simulink model "linear"  (R2016b)
settings: Solver=VariableStepAuto  StartTime=0.0  StopTime=100.0  RelTol=1e-3
undefined symbols (not defined in the file or in its folder): magnitude
libraries: simulink x1
settings Model: Creator=tangxiaoli  LastModifiedBy=tangxiaoli

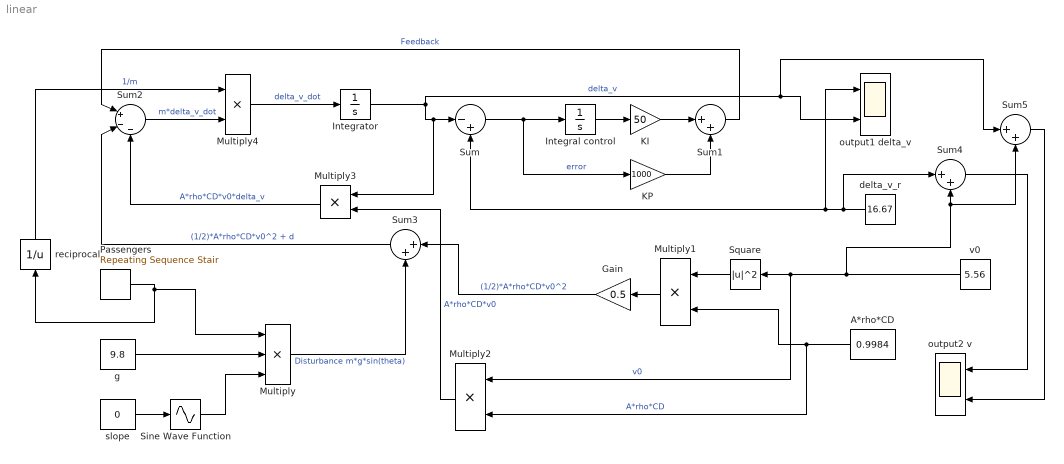
== system linear ==
  " Square" : Math  Operator=magnitude^2  SaturateOnIntegerOverflow=on
  A*rho*CD : Constant  Value=0.9984
  Gain : Gain  Gain=0.5
  Integral control : Integrator
  Integrator : Integrator
  KI : Gain  Gain=50
  KP : Gain  Gain=1000
  Multiply : Product  Inputs=***
  Multiply{1..4} (4 alike) : Product  Inputs=**
  Passengers : simulink/Sources/Repeating Sequence Stair  OutValues=[1600 1662 1724 1786 1848 1910].'  tsamp=20  OutMin=[]  OutMax=[]  OutDataTypeStr=double  OutputDataTypeScalingMode=double  OutDataType=fixdt(0,8)  ConRadixGroup=Best Precision: Vector-wise  OutScaling=2^-12
  Sine Wave Function : Sin  TimeSource=Use external signal  SampleTime=0
  Sum : Sum  Inputs=|-+
  Sum{1,3..5} (4 alike) : Sum  Inputs=|++
  Sum2 : Sum  Inputs=|+--
  delta_v_r : Constant  Value=16.67
  g : Constant  Value=9.8
  output1 delta_v : Scope  NumInputPorts=2
  output2 v : Scope  NumInputPorts=2
  reciprocal : Math  Operator=reciprocal  SaturateOnIntegerOverflow=on
  slope : Constant  Value=0
  v0 : Constant  Value=5.56
  wires:
  Multiply4/1 -> Integrator/1  "delta_v_dot"
  Integrator/1 -> Multiply3/1, Sum/1, Sum5/1, output1 delta_v/2  "delta_v"
  Integral control/1 -> KI/1
  Sum/1 -> KP/1, Integral control/1  "error"
  KI/1 -> Sum1/1
  KP/1 -> Sum1/2
  Sum2/1 -> Multiply4/2  "m*delta_v_dot"
  Sum1/1 -> Sum2/1  "Feedback"
  delta_v_r/1 -> Sum4/1, output1 delta_v/1, Sum/2
  Sum3/1 -> Sum2/2  "(1/2)*A*rho*CD*v0^2 + d"
  Gain/1 -> Sum3/1  "(1/2)*A*rho*CD*v0^2"
  Passengers/1 -> reciprocal/1, Multiply/1
  g/1 -> Multiply/2
  Sine Wave Function/1 -> Multiply/3
  Multiply/1 -> Sum3/2  "Disturbance m*g*sin(theta)"
  v0/1 -> Multiply2/1, " Square"/1, Sum5/2, Sum4/2  "v0"
  " Square"/1 -> Multiply1/1
  A*rho*CD/1 -> Multiply2/2, Multiply1/2  "A*rho*CD"
  Multiply1/1 -> Gain/1
  Multiply2/1 -> Multiply3/2  "A*rho*CD*v0"
  Multiply3/1 -> Sum2/3  "A*rho*CD*v0*delta_v"
  Sum4/1 -> output2 v/1
  Sum5/1 -> output2 v/2
  reciprocal/1 -> Multiply4/1  "1/m"
  slope/1 -> Sine Wave Function/1
